simulink model "System5"  (R2018b)
settings: Solver=VariableStepAuto  StartTime=0.0  StopTime=10.0  RelTol=1e-3
libraries: cstblocks x2
settings Model: Creator=Abraham Pérez  LastModifiedBy=Abraham Pérez

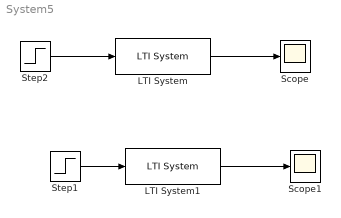
== system System5 ==
  LTI System : cstblocks/LTI System  sys=g5a  IC=[]
  LTI System1 : cstblocks/LTI System  sys=g5b  IC=[]
  Scope : Scope
  Scope1 : Scope
  Step1 : Step  Time=0  Before=4.7  After=4.7  SampleTime=0
  Step2 : Step  Time=0  Before=3.5  After=3.5  SampleTime=0
  wires:
  Step1/1 -> LTI System1/1
  LTI System/1 -> Scope/1
  LTI System1/1 -> Scope1/1
  Step2/1 -> LTI System/1
